simulink model "zero_moment_direction_ctrl"  (R2018b)
settings: Solver=VariableStepAuto  StartTime=0.0  StopTime=40  RelTol=1e-3
values from neighbouring files (symbols this model uses):
  alpha_0 = alpha    (= 0.237364778271)    [IdealParameter.m]    (also in Parameter.m = alpha; ParameterIdeal.m = alpha*1.01; ParameterVIVE.m = alpha*1.01; ParameterVO.m = alpha*1.01)
  angular_noise = 0    [IdealParameter.m]    (also in Parameter.m = 0.5; ParameterIdeal.m; ParameterVIVE.m; ParameterVO.m)
  b_0 = b*1.15    (= 1.265e-06)    [IdealParameter.m]    (also in Parameter.m = 8.944e-07; ParameterIdeal.m; ParameterVIVE.m; ParameterVO.m)
  beta_0 = beta    (= 0)    [IdealParameter.m]    (also in Parameter.m = beta; ParameterIdeal.m = beta*0.99; ParameterVIVE.m = beta*0.99; ParameterVO.m = beta*0.99)
  g_0 = g*0.99    (= 9.7119)    [IdealParameter.m]    (also in Parameter.m = 9.81; ParameterIdeal.m = 9.81; ParameterVIVE.m = 9.81; ParameterVO.m = 9.81)
  IB = [Ixx 0 0; 0 Iyy 0; 0 0 Izz]    [IdealParameter.m]    (also in ParLuk11.m; Parameter.m; ParameterIdeal.m; ParameterVIVE.m)
  IB_0 = IB*1.07    [IdealParameter.m]    (also in Parameter.m = IB; ParameterIdeal.m; ParameterVIVE.m; ParameterVO.m)
  K_0 = Ts/(T_rotor_0+Ts)    (= 0.0384615384615)    [IdealParameter.m]    (also in Parameter.m; ParameterIdeal.m; ParameterVIVE.m = 0.0350877192982; ParameterVO.m = 0.214285714286)
  k_0 = k*1.16    (= 6.496e-05)    [IdealParameter.m]    (also in Parameter.m = 4.472e-05; ParameterIdeal.m; ParameterVIVE.m = 5.9508e-05; ParameterVO.m)
  K_ad = 4    [Parameter.m]
  K_ap = 2    [Parameter.m]
  K_pd = 8    [Parameter.m]
  K_pp = 6    [Parameter.m]
  K_z = 5    [Parameter.m]
  L_0 = L*1.02    (= 0.408)    [IdealParameter.m]    (also in Parameter.m = 0.4; ParameterIdeal.m; ParameterVIVE.m = 0.612; ParameterVO.m)
  m_0 = m*1.03    (= 2.575)    [IdealParameter.m]    (also in Parameter.m = 4.85; ParameterIdeal.m = 4.9955; ParameterVIVE.m = 4.52994; ParameterVO.m = 4.9955)
  omega_noise = 0    [IdealParameter.m]    (also in Parameter.m = 0.0027; ParameterIdeal.m; ParameterVIVE.m; ParameterVO.m)
  p_noise = 0    [IdealParameter.m]    (also in Parameter.m = 0.00064; ParameterIdeal.m; ParameterVIVE.m; ParameterVO.m)
  rot_vel_max = (6300 * pi/30)^2    (= 435249.554088)    [Parameter.m]    (also in ParameterVIVE.m = 356292.718879; Parameter_old.m)
  rot_vel_min = 0    [Parameter.m]    (also in ParameterVIVE.m; Parameter_old.m)
  T_delay = 0    [IdealParameter.m]    (also in Parameter.m = 0.04; ParameterIdeal.m; ParameterVIVE.m = 0.04; ParameterVO.m = 0.1)
  T_rotor = 0.1    [IdealParameter.m]    (also in Parameter.m; ParameterIdeal.m; ParameterVIVE.m; ParameterVO.m)
  Ts = 1/250    (= 0.004)    [IdealParameter.m]    (also in Parameter.m; ParameterIdeal.m; ParameterVIVE.m; ParameterVO.m = 0.03)
  v_noise = 0    [IdealParameter.m]    (also in Parameter.m = 0.0014; ParameterIdeal.m; ParameterVIVE.m; ParameterVO.m)
  z_p_0 = T_rotor_0/(T_rotor_0+Ts)    (= 0.961538461538)    [IdealParameter.m]    (also in Parameter.m; ParameterIdeal.m; ParameterVIVE.m = 0.964912280702; ParameterVO.m = 0.785714285714)
libraries: simulink x7, vrlib x2
settings Model: Creator=HaloCao  LastModifiedBy=HaloCao

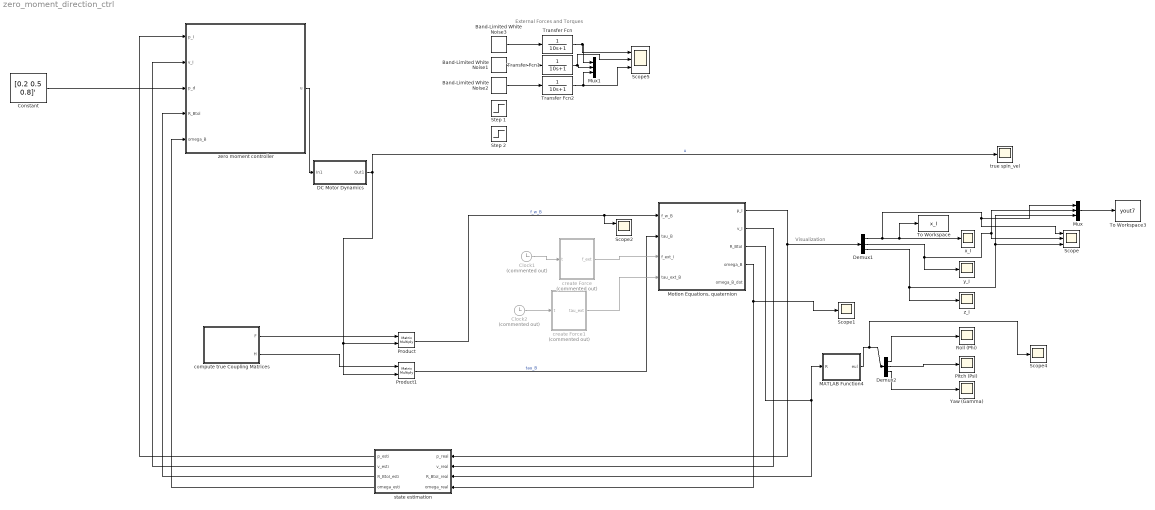
== system zero_moment_direction_ctrl ==
  note: Visualization
  note: External Forces and Torques
  Band-Limited White Noise1 : simulink/Sources/Band-Limited White Noise  Cov=1  Ts=0.1  seed=[23342]  VectorParams1D=off
  Band-Limited White Noise2 : simulink/Sources/Band-Limited White Noise  Cov=1  Ts=0.1  seed=[23441]  VectorParams1D=off
  Band-Limited White Noise3 : simulink/Sources/Band-Limited White Noise  Cov=1  Ts=0.1  seed=[23342]  VectorParams1D=off
  Clock1 : Clock  Commented=on
  Clock2 : Clock  Commented=on
  Constant : Constant  Value="[0.2  0.5 0.8]'"
  "DC Motor Dynamics " : Subsystem  TreatAsAtomicUnit=on
  Demux1 : Demux  Outputs=3
  Demux2 : Demux  Outputs=3
  MATLAB Function4 : MATLAB Function  TreatAsAtomicUnit=on
  "Motion Equations, quaternion" : Subsystem
  Mux : Mux  Inputs=3
  Mux1 : Mux  Inputs=3
  Pitch (Psi) : Scope
  Product : Product  Multiplication=Matrix(*)
  Product1 : Product  Multiplication=Matrix(*)
  Roll (Phi) : Scope
  Scope : Scope  NumInputPorts=3
  Scope1 : Scope
  Scope2 : Scope  NumInputPorts=2
  Scope4 : Scope
  Scope5 : Scope  NumInputPorts=3
  Step 1 : Step  Before=[0;0;0]  After=[10;1;1]  SampleTime=0  VectorParams1D=off
  Step 2 : Step  Before=[0;0;0]  After=[5;1;1]  SampleTime=0  VectorParams1D=off
  To Workspace : ToWorkspace  VariableName=x_I  SaveFormat=Timeseries  SampleTime=-1
  To Workspace3 : ToWorkspace  VariableName=yout7  SampleTime=-1
      settings: Save2DSignal=2-D array (concatenate along first dimension)
  Transfer Fcn : TransferFcn  Denominator=[10 1]
  Transfer Fcn1 : TransferFcn  Denominator=[10 1]
  Transfer Fcn2 : TransferFcn  Denominator=[10 1]
  Yaw (Gamma) : Scope
  compute true Coupling Matrices : Subsystem
  create Force : MATLAB Function  Commented=on  TreatAsAtomicUnit=on
  create Force1 : MATLAB Function  Commented=on  TreatAsAtomicUnit=on
  state estimation : Subsystem
  true spin_vel : Scope
  x_I : Scope
  y_I : Scope
  z_I : Scope
  zero moment controller : Subsystem
  wires:
  zero moment controller/1(u) -> "DC Motor Dynamics "/1(In1)
  "Motion Equations, quaternion"/1(p_I) -> state estimation/1(p_real), Demux1/1
  Demux2/2 -> Pitch (Psi)/1
  Demux1/2 -> Mux/2, Scope/2, y_I/1
  Product1/1 -> "Motion Equations, quaternion"/2(tau_B)  "tau_B"
  Demux2/3 -> Yaw (Gamma)/1
  "Motion Equations, quaternion"/2(v_I) -> state estimation/2(v_real)
  MATLAB Function4/1(eul) -> Scope4/1, Demux2/1
  Demux1/3 -> Mux/3, Scope/3, z_I/1
  "Motion Equations, quaternion"/4(omega_B) -> state estimation/4(omega_real), Scope1/1
  Demux2/1 -> Roll (Phi)/1
  "Motion Equations, quaternion"/3(R_BtoI) -> state estimation/3(R_BtoI_real), MATLAB Function4/1(R)
  Constant/1 -> zero moment controller/3(p_d)
  Demux1/1 -> Mux/1, Scope/1, To Workspace/1, x_I/1
  Clock1/1 -> create Force/1(t)
  compute true Coupling Matrices/1(F) -> Product/1
  compute true Coupling Matrices/2(H) -> Product1/1
  "DC Motor Dynamics "/1(Out1) -> Product1/2, Product/2, true spin_vel/1  "u"
  Product/1 -> Scope2/1, "Motion Equations, quaternion"/1("f_w_B ")  "f_w_B"
  Mux/1 -> To Workspace3/1
  state estimation/3(R_BtoI_esti) -> zero moment controller/4(R_Btol)
  state estimation/4(omega_esti) -> zero moment controller/5(omega_B)
  state estimation/2(v_esti) -> zero moment controller/2(v_I)
  state estimation/1(p_esti) -> zero moment controller/1(p_I)
  Clock2/1 -> create Force1/1(t)
  Transfer Fcn1/1 -> Scope5/2, Mux1/2
  Band-Limited White Noise3/1 -> Transfer Fcn/1
  Transfer Fcn2/1 -> Scope5/3, Mux1/3
  Band-Limited White Noise2/1 -> Transfer Fcn2/1
  Band-Limited White Noise1/1 -> Transfer Fcn1/1
  Transfer Fcn/1 -> Scope5/1, Mux1/1
  create Force1/1(tau_ext) -> "Motion Equations, quaternion"/4(tau_ext_B)
  create Force/1(f_ext) -> "Motion Equations, quaternion"/3(f_ext_I)

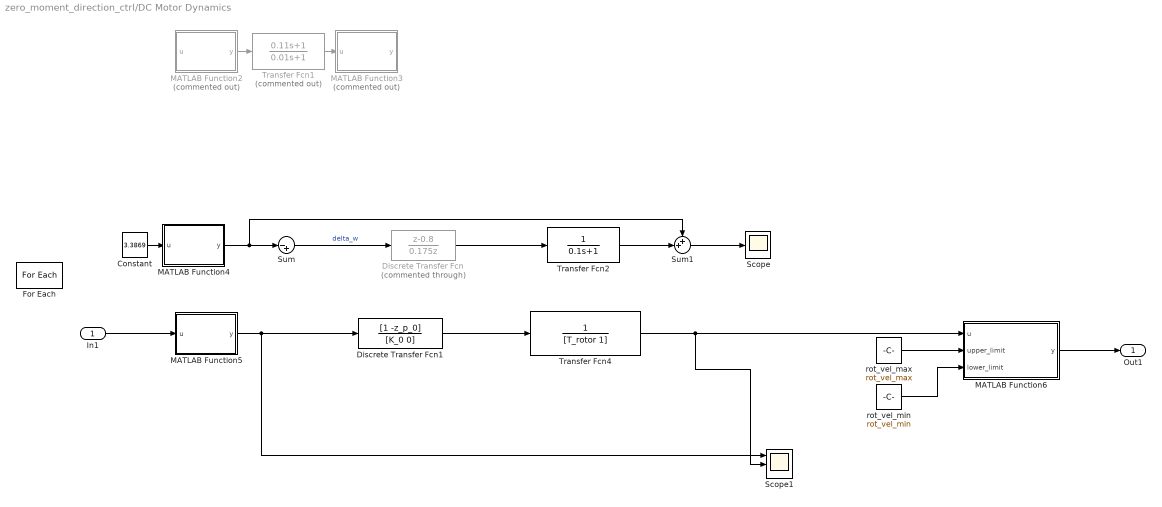
== system zero_moment_direction_ctrl/DC Motor Dynamics  ==
  In1 : Inport  Partition=on  PartitionDimension=1  PartitionWidth=1  PartitionOffset=0
  Constant : Constant  Value=3.3869
  Discrete Transfer Fcn : DiscreteTransferFcn  Commented=through  Numerator=[1 -0.8]  Denominator=[0.175 0]  SampleTime=Ts
  Discrete Transfer Fcn1 : DiscreteTransferFcn  Numerator=[1 -z_p_0]  Denominator=[K_0 0]  InitialStates=274  SampleTime=Ts
  For Each : ForEach  DisableCoverage=on  IndexMode=One-based
  MATLAB Function2 : MATLAB Function  Commented=on  TreatAsAtomicUnit=on
  MATLAB Function3 : MATLAB Function  Commented=on  TreatAsAtomicUnit=on
  MATLAB Function4 : MATLAB Function  TreatAsAtomicUnit=on
  MATLAB Function5 : MATLAB Function  TreatAsAtomicUnit=on  SystemSampleTime=Ts
  MATLAB Function6 : MATLAB Function  TreatAsAtomicUnit=on
  Scope : Scope
  Scope1 : Scope  NumInputPorts=3
  Sum : Sum  Inputs=|-+
  Sum1 : Sum  Inputs=++|
  Transfer Fcn1 : TransferFcn  Commented=on  Numerator=[0.11 1]  Denominator=[0.01 1]
  Transfer Fcn2 : TransferFcn  Denominator=[0.1 1]
  Transfer Fcn4 : TransferFcn  Denominator=[T_rotor 1]
  rot_vel_max : Constant  Value=rot_vel_max
  rot_vel_min : Constant  Value=rot_vel_min
  Out1 : Outport  ConcatenationDimension=1
  wires:
  Transfer Fcn1/1 -> MATLAB Function3/1(u)
  MATLAB Function2/1(y) -> Transfer Fcn1/1
  Constant/1 -> MATLAB Function4/1(u)
  MATLAB Function4/1(y) -> Sum1/1, Sum/1
  Sum/1 -> Discrete Transfer Fcn/1  "delta_w"
  In1/1 -> MATLAB Function5/1(u)
  MATLAB Function5/1(y) -> Discrete Transfer Fcn1/1, Scope1/1
  Discrete Transfer Fcn/1 -> Transfer Fcn2/1
  Transfer Fcn2/1 -> Sum1/2
  MATLAB Function6/1(y) -> Out1/1
  Sum1/1 -> Scope/1
  Discrete Transfer Fcn1/1 -> Transfer Fcn4/1
  Transfer Fcn4/1 -> Scope1/2, MATLAB Function6/1(u)
  rot_vel_max/1 -> MATLAB Function6/2(upper_limit)
  rot_vel_min/1 -> MATLAB Function6/3(lower_limit)

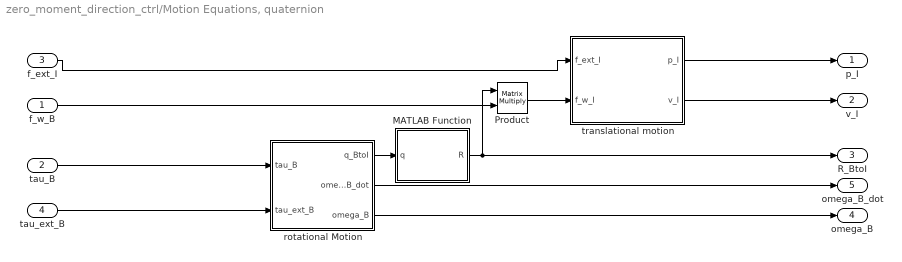
== system zero_moment_direction_ctrl/Motion Equations, quaternion ==
  "f_w_B " : Inport
  tau_B : Inport  Port=2
  f_ext_I : Inport  Port=3
  tau_ext_B : Inport  Port=4
  MATLAB Function : MATLAB Function  TreatAsAtomicUnit=on
  Product : Product  Multiplication=Matrix(*)
  rotational Motion : Subsystem
  translational motion : Subsystem
  p_I : Outport
  v_I : Outport  Port=2
  R_BtoI : Outport  Port=3
  omega_B : Outport  Port=4
  omega_B_dot : Outport  Port=5
  wires:
  f_ext_I/1 -> translational motion/1(f_ext_I)
  translational motion/1(p_I) -> p_I/1
  translational motion/2(v_I) -> v_I/1
  Product/1 -> translational motion/2(f_w_I)
  tau_B/1 -> rotational Motion/1(tau_B)
  tau_ext_B/1 -> rotational Motion/2(tau_ext_B)
  rotational Motion/2(omega_B_dot) -> omega_B_dot/1
  rotational Motion/3(omega_B) -> omega_B/1
  "f_w_B "/1 -> Product/2
  rotational Motion/1(q_BtoI) -> MATLAB Function/1(q)
  MATLAB Function/1(R) -> Product/1, R_BtoI/1

== system zero_moment_direction_ctrl/compute true Coupling Matrices ==
  Constant : Constant  Value=alpha_0
  Constant2 : Constant  Value=beta_0
  Constant3 : Constant  Value=k_0
  Constant4 : Constant  Value=L_0
  Constant5 : Constant  Value=b_0
  MATLAB Function5 : MATLAB Function  TreatAsAtomicUnit=on
  MATLAB Function6 : MATLAB Function  TreatAsAtomicUnit=on
  F : Outport
  H : Outport  Port=2
  wires:
  MATLAB Function5/6(e_r6) -> MATLAB Function6/6(e_r6)
  Constant4/1 -> MATLAB Function6/9(L)
  MATLAB Function5/2(e_r2) -> MATLAB Function6/2(e_r2)
  MATLAB Function5/3(e_r3) -> MATLAB Function6/3(e_r3)
  MATLAB Function5/4(e_r4) -> MATLAB Function6/4(e_r4)
  MATLAB Function5/1(e_r1) -> MATLAB Function6/1(e_r1)
  MATLAB Function5/5(e_r5) -> MATLAB Function6/5(e_r5)
  Constant3/1 -> MATLAB Function6/8(k)
  Constant2/1 -> MATLAB Function5/2(beta)
  Constant/1 -> MATLAB Function5/1(alpha)
  Constant5/1 -> MATLAB Function6/7(b)
  MATLAB Function6/2(H) -> H/1
  MATLAB Function6/1(F) -> F/1

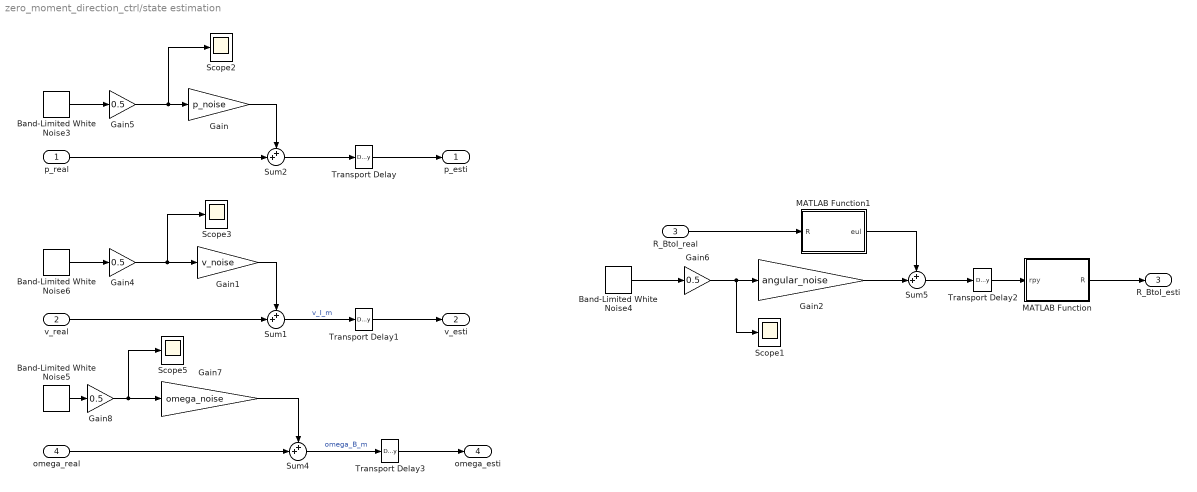
== system zero_moment_direction_ctrl/state estimation ==
  p_real : Inport
  v_real : Inport  Port=2
  R_BtoI_real : Inport  Port=3
  omega_real : Inport  Port=4
  Band-Limited White Noise3 : simulink/Sources/Band-Limited White Noise  Cov=[0.01; 0.01; 0.01]  Ts=Ts  seed=[22352; 29655; 12541]  VectorParams1D=off
  Band-Limited White Noise4 : simulink/Sources/Band-Limited White Noise  Cov=[0.01; 0.01; 0.01]  Ts=Ts  seed=[11351; 22653; 52546]  VectorParams1D=off
  Band-Limited White Noise5 : simulink/Sources/Band-Limited White Noise  Cov=[0.01; 0.01; 0.01]  Ts=Ts  seed=[12451; 82653; 82546]  VectorParams1D=off
  Band-Limited White Noise6 : simulink/Sources/Band-Limited White Noise  Cov=[0.01; 0.01; 0.01]  Ts=Ts  seed=[22351; 29653; 12546]  VectorParams1D=off
  Gain : Gain  Gain=p_noise
  Gain1 : Gain  Gain=v_noise
  Gain2 : Gain  Gain=angular_noise
  Gain{4..6,8} (4 alike) : Gain  Gain=0.5
  Gain7 : Gain  Gain=omega_noise
  MATLAB Function : MATLAB Function  TreatAsAtomicUnit=on
  MATLAB Function1 : MATLAB Function  TreatAsAtomicUnit=on
  Scope{1..3,5} (4 alike) : Scope
  Sum{1..2,4..5} (4 alike) : Sum  Inputs=++|
  Transport Delay{,1..3} (4 alike) : TransportDelay  DelayTime=T_delay  InitialOutput=[0;0;0]
  p_esti : Outport
  v_esti : Outport  Port=2
  R_BtoI_esti : Outport  Port=3
  omega_esti : Outport  Port=4
  wires:
  R_BtoI_real/1 -> MATLAB Function1/1(R)
  p_real/1 -> Sum2/2
  Transport Delay/1 -> p_esti/1
  Sum4/1 -> Transport Delay3/1  "omega_B_m"
  Gain/1 -> Sum2/1
  Gain1/1 -> Sum1/1
  Sum2/1 -> Transport Delay/1
  Sum1/1 -> Transport Delay1/1  "v_I_m"
  MATLAB Function1/1(eul) -> Sum5/1
  Sum5/1 -> Transport Delay2/1
  Gain2/1 -> Sum5/2
  Transport Delay2/1 -> MATLAB Function/1(rpy)
  v_real/1 -> Sum1/2
  omega_real/1 -> Sum4/2
  MATLAB Function/1(R) -> R_BtoI_esti/1
  Transport Delay1/1 -> v_esti/1
  Gain5/1 -> Scope2/1, Gain/1
  Band-Limited White Noise3/1 -> Gain5/1
  Gain4/1 -> Gain1/1, Scope3/1
  Band-Limited White Noise6/1 -> Gain4/1
  Band-Limited White Noise5/1 -> Gain8/1
  Gain8/1 -> Scope5/1, Gain7/1
  Gain6/1 -> Scope1/1, Gain2/1
  Band-Limited White Noise4/1 -> Gain6/1
  Transport Delay3/1 -> omega_esti/1
  Gain7/1 -> Sum4/1

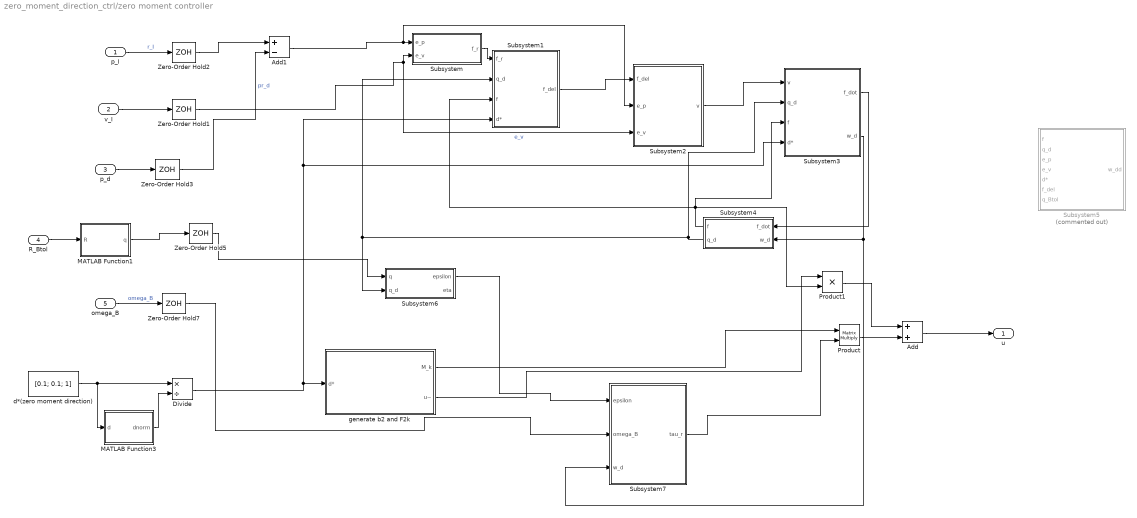
== system zero_moment_direction_ctrl/zero moment controller ==
  p_I : Inport
  v_I : Inport  Port=2
  p_d : Inport  Port=3
  R_Btol : Inport  Port=4
  omega_B : Inport  Port=5
  Add : Sum
  Add1 : Sum  Inputs=+-
  Divide : Product  Inputs=*/
  MATLAB Function1 : MATLAB Function  TreatAsAtomicUnit=on
  MATLAB Function3 : MATLAB Function  TreatAsAtomicUnit=on
  Product : Product  Multiplication=Matrix(*)
  Product1 : Product
  Subsystem : Subsystem
  Subsystem1 : Subsystem
  Subsystem2 : Subsystem
  Subsystem3 : Subsystem
  Subsystem4 : Subsystem
  Subsystem5 : Subsystem  Commented=on
  Subsystem6 : Subsystem
  Subsystem7 : Subsystem
  Zero-Order Hold{1..3,5,7} (5 alike) : ZeroOrderHold  SampleTime=Ts
  d*(zero moment direction) : Constant  Value=[0.1; 0.1; 1]
  generate b2 and F2k : Subsystem
  u : Outport
  wires:
  p_d/1 -> Zero-Order Hold3/1
  p_I/1 -> Zero-Order Hold2/1  "r_I"
  Zero-Order Hold5/1 -> Subsystem6/1(q)
  omega_B/1 -> Zero-Order Hold7/1  "omega_B"
  Zero-Order Hold1/1 -> Subsystem/2(e_v), Subsystem2/3(e_v)  "e_v"
  Subsystem/1(f_r) -> Subsystem1/1(f_r)
  Subsystem1/1(f_del) -> Subsystem2/1(f_del)
  Subsystem2/1(v) -> Subsystem3/1(v)
  Subsystem3/1(f_dot) -> Subsystem4/1(f_dot)
  Subsystem3/2(w_d) -> Subsystem7/3(w_d), Subsystem4/2(w_d)
  Subsystem4/1(f) -> Subsystem3/3(f), Product1/2, Subsystem1/3(f)
  Subsystem7/1(tau_r) -> Product/2
  generate b2 and F2k/1(M_k) -> Product/1
  Add/1 -> u/1
  generate b2 and F2k/2(u~) -> Product1/1
  Product/1 -> Add/2
  Product1/1 -> Add/1
  Subsystem6/1(epsilon) -> Subsystem7/1(epsilon)
  v_I/1 -> Zero-Order Hold1/1
  Zero-Order Hold3/1 -> Add1/2  "pr_d"
  Zero-Order Hold2/1 -> Add1/1
  MATLAB Function3/1(dnorm) -> Divide/2
  d*(zero moment direction)/1 -> MATLAB Function3/1(d), Divide/1
  Divide/1 -> Subsystem3/4(d*), Subsystem1/4(d*), generate b2 and F2k/1(d*)
  Add1/1 -> Subsystem2/2(e_p), Subsystem/1(e_p)
  Subsystem4/2(q_d) -> Subsystem1/2(q_d), Subsystem6/2(q_d), Subsystem3/2(q_d)
  Zero-Order Hold7/1 -> Subsystem7/2(omega_B)
  R_Btol/1 -> MATLAB Function1/1(R)
  MATLAB Function1/1(q) -> Zero-Order Hold5/1

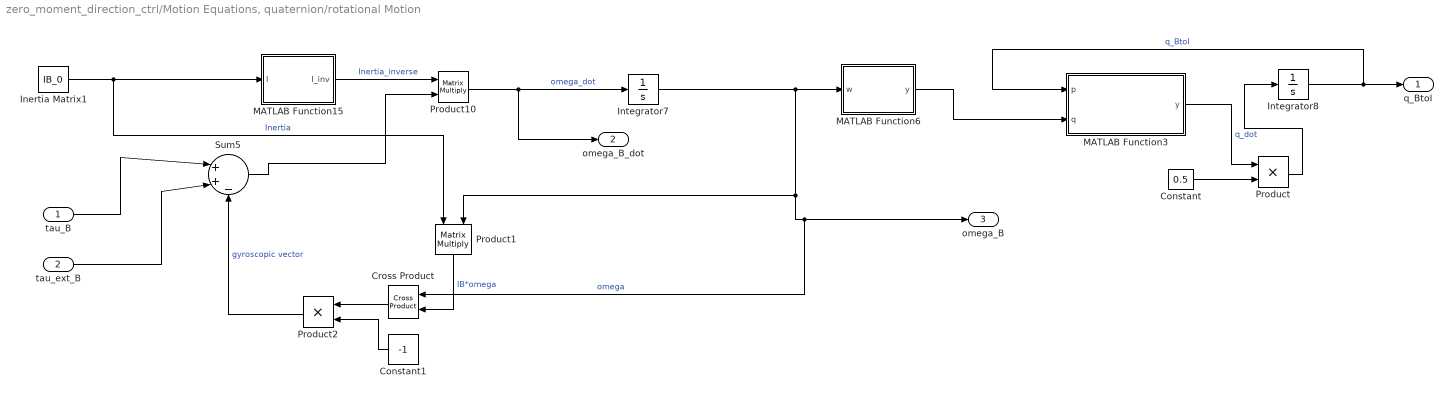
== system zero_moment_direction_ctrl/Motion Equations, quaternion/rotational Motion ==
  tau_B : Inport
  tau_ext_B : Inport  Port=2
  Constant : Constant  Value=0.5
  Constant1 : Constant  Value=-1
  Cross Product : vrlib/Utilities/Cross Product
      settings: SourceProductBaseCode=VR
  Inertia Matrix1 : Constant  Value=IB_0  VectorParams1D=off
  Integrator7 : Integrator  InitialCondition=[0 0 0]'
  Integrator8 : Integrator  InitialCondition=[0 0 0 1]'
  MATLAB Function15 : MATLAB Function  TreatAsAtomicUnit=on
  MATLAB Function3 : MATLAB Function  TreatAsAtomicUnit=on
  MATLAB Function6 : MATLAB Function  TreatAsAtomicUnit=on
  Product : Product
  Product1 : Product  Multiplication=Matrix(*)
  Product10 : Product  Multiplication=Matrix(*)
  Product2 : Product
  Sum5 : Sum  Inputs=|++-
  q_BtoI : Outport
  omega_B_dot : Outport  Port=2
  omega_B : Outport  Port=3
  wires:
  Product10/1 -> omega_B_dot/1, Integrator7/1  "omega_dot"
  tau_B/1 -> Sum5/1
  Integrator7/1 -> Product1/2, Cross Product/1, omega_B/1, MATLAB Function6/1(w)  "omega"
  tau_ext_B/1 -> Sum5/2
  Inertia Matrix1/1 -> Product1/1, MATLAB Function15/1(I)  "Inertia"
  Sum5/1 -> Product10/2
  MATLAB Function15/1(I_inv) -> Product10/1  "Inertia_inverse"
  Integrator8/1 -> MATLAB Function3/1(p), q_BtoI/1  "q_BtoI"
  Product2/1 -> Sum5/3  "gyroscopic vector"
  Product1/1 -> Cross Product/2  "IB*omega"
  Constant/1 -> Product/2
  Product/1 -> Integrator8/1
  MATLAB Function3/1(y) -> Product/1  "q_dot"
  MATLAB Function6/1(y) -> MATLAB Function3/2(q)
  Cross Product/1 -> Product2/1
  Constant1/1 -> Product2/2

== system zero_moment_direction_ctrl/Motion Equations, quaternion/translational motion ==
  f_ext_I : Inport
  f_w_I : Inport  Port=2
  Constant1 : Constant  Value=[0 0 g_0]'  VectorParams1D=off
  Gain1 : Gain  Gain=m_0
  Gain4 : Gain  Gain=1/m_0
  Integrator2 : Integrator  InitialCondition=[0;0;0]
  Integrator3 : Integrator  InitialCondition=[0 0 0]'
  Sum : Sum  Inputs=++-
  p_I : Outport
  v_I : Outport  Port=2
  wires:
  Sum/1 -> Gain4/1
  f_ext_I/1 -> Sum/1
  Gain4/1 -> Integrator2/1  "a_I"
  Integrator2/1 -> v_I/1, Integrator3/1  "v_I"
  Gain1/1 -> Sum/3  "gravity"
  Constant1/1 -> Gain1/1
  Integrator3/1 -> p_I/1  "p_I"
  f_w_I/1 -> Sum/2

== system zero_moment_direction_ctrl/zero moment controller/Subsystem ==
  e_p : Inport
  e_v : Inport  Port=2
  Constant1 : Constant  Value=[0 0 g_0]'  VectorParams1D=off
  Gain1 : Gain  Gain=m_0
  K_pd : Constant  Value=K_pd
  K_pp : Constant  Value=K_pp
  Product : Product
  Product1 : Product
  Sum : Sum  Inputs=-+-
  f_r : Outport
  wires:
  Product/1 -> Sum/1
  Constant1/1 -> Gain1/1
  Gain1/1 -> Sum/2  "gravity"
  K_pp/1 -> Product/1
  e_p/1 -> Product/2
  K_pd/1 -> Product1/1
  e_v/1 -> Product1/2
  Product1/1 -> Sum/3
  Sum/1 -> f_r/1

== system zero_moment_direction_ctrl/zero moment controller/Subsystem1 ==
  f_r : Inport
  q_d : Inport  Port=2
  f : Inport  Port=3
  d* : Inport  Port=4
  MATLAB Function1 : MATLAB Function  TreatAsAtomicUnit=on
  Minus : Sum  Inputs=-+
  Product : Product  Multiplication=Matrix(*)
  Product1 : Product
  f_del : Outport
  wires:
  d*/1 -> Product/2
  Product/1 -> Product1/1
  f/1 -> Product1/2
  Product1/1 -> Minus/2
  f_r/1 -> Minus/1
  Minus/1 -> f_del/1
  MATLAB Function1/1(R) -> Product/1
  q_d/1 -> MATLAB Function1/1(q)

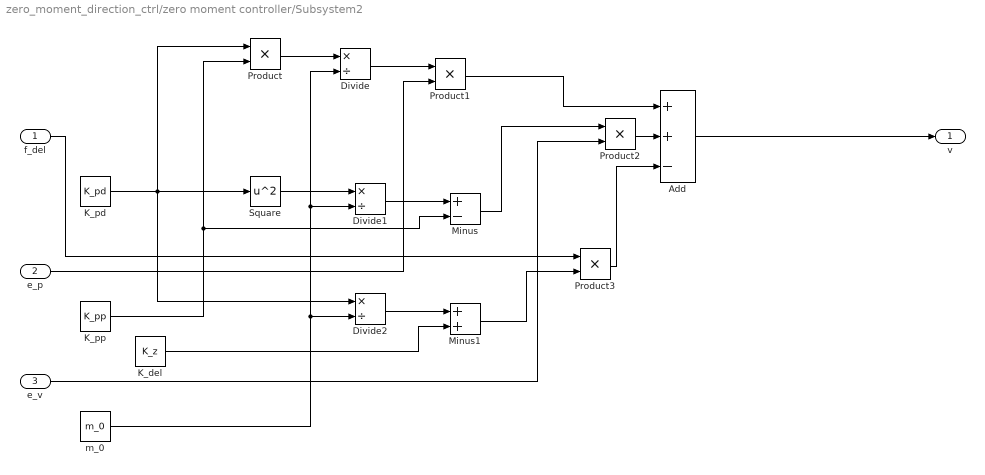
== system zero_moment_direction_ctrl/zero moment controller/Subsystem2 ==
  f_del : Inport
  e_p : Inport  Port=2
  e_v : Inport  Port=3
  Add : Sum  Inputs=++-
  Divide : Product  Inputs=*/
  Divide1 : Product  Inputs=*/
  Divide2 : Product  Inputs=*/
  K_del : Constant  Value=K_z
  K_pd : Constant  Value=K_pd
  K_pp : Constant  Value=K_pp
  Minus : Sum  Inputs=+-
  Minus1 : Sum
  Product{,1..3} (4 alike) : Product
  Square : Math  Operator=square  SaturateOnIntegerOverflow=on
  m_0 : Constant  Value=m_0
  v : Outport
  wires:
  K_pd/1 -> Product/1, Divide2/1, Square/1
  K_pp/1 -> Minus/2, Product/2
  Product/1 -> Divide/1
  m_0/1 -> Divide2/2, Divide1/2, Divide/2
  Divide/1 -> Product1/1
  e_p/1 -> Product1/2
  Product1/1 -> Add/1
  Square/1 -> Divide1/1
  Divide1/1 -> Minus/1
  Minus/1 -> Product2/1
  e_v/1 -> Product2/2
  Product2/1 -> Add/2
  Divide2/1 -> Minus1/1
  K_del/1 -> Minus1/2
  Product3/1 -> Add/3
  Minus1/1 -> Product3/2
  f_del/1 -> Product3/1
  Add/1 -> v/1

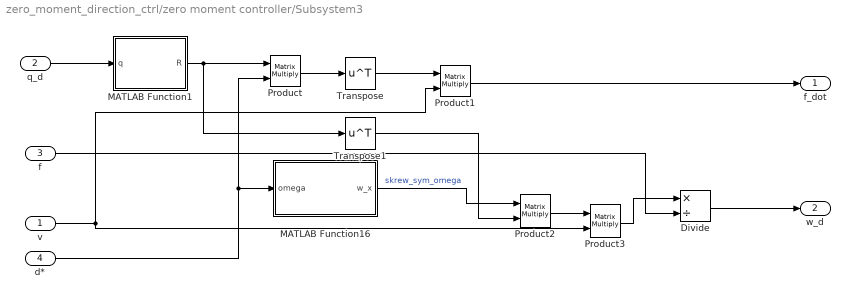
== system zero_moment_direction_ctrl/zero moment controller/Subsystem3 ==
  v : Inport
  q_d : Inport  Port=2
  f : Inport  Port=3
  d* : Inport  Port=4
  Divide : Product  Inputs=*/
  MATLAB Function1 : MATLAB Function  TreatAsAtomicUnit=on
  MATLAB Function16 : MATLAB Function  TreatAsAtomicUnit=on
  Product{,1..3} (4 alike) : Product  Multiplication=Matrix(*)
  Transpose : Math  Operator=transpose  SaturateOnIntegerOverflow=on
  Transpose1 : Math  Operator=transpose  SaturateOnIntegerOverflow=on
  f_dot : Outport
  w_d : Outport  Port=2
  wires:
  d*/1 -> Product/2, MATLAB Function16/1(omega)
  Product/1 -> Transpose/1
  Transpose/1 -> Product1/1
  v/1 -> Product1/2, Product3/2
  Product1/1 -> f_dot/1
  f/1 -> Divide/2
  Divide/1 -> w_d/1
  MATLAB Function16/1(w_x) -> Product2/1  "skrew_sym_omega"
  Transpose1/1 -> Product2/2
  q_d/1 -> MATLAB Function1/1(q)
  MATLAB Function1/1(R) -> Transpose1/1, Product/1
  Product2/1 -> Product3/1
  Product3/1 -> Divide/1

== system zero_moment_direction_ctrl/zero moment controller/Subsystem4 ==
  f_dot : Inport
  w_d : Inport  Port=2
  Constant : Constant  Value=0.5
  Integrator : Integrator  InitialCondition=47.5
  Integrator1 : Integrator  InitialCondition=[0 0 0 1]'
  MATLAB Function : MATLAB Function  TreatAsAtomicUnit=on
  MATLAB Function1 : MATLAB Function  TreatAsAtomicUnit=on
  Product : Product
  f : Outport
  q_d : Outport  Port=2
  wires:
  Integrator/1 -> f/1
  Integrator1/1 -> MATLAB Function/1(p), q_d/1
  w_d/1 -> MATLAB Function1/1(w)
  MATLAB Function/1(y) -> Product/1
  Constant/1 -> Product/2
  MATLAB Function1/1(y) -> MATLAB Function/2(q)
  f_dot/1 -> Integrator/1
  Product/1 -> Integrator1/1

== system zero_moment_direction_ctrl/zero moment controller/Subsystem5 ==
  f : Inport
  q_d : Inport  Port=2
  e_p : Inport  Port=3
  e_v : Inport  Port=4
  d* : Inport  Port=5
  f_del : Inport  Port=6
  q_Btol : Inport  Port=7
  MATLAB Function : MATLAB Function  TreatAsAtomicUnit=on
  Product2 : Product  Multiplication=Matrix(*)
  teil1 : Subsystem
  teil2 : Subsystem
  w_dd : Outport
  wires:
  q_d/1 -> teil2/2(q_d), teil1/2(q_d)
  f/1 -> teil2/1(f), teil1/1(f)
  d*/1 -> teil1/3(d*), teil2/5(d*)
  teil1/1(Out1) -> Product2/1
  f_del/1 -> teil2/6(f_del)
  e_p/1 -> teil2/3(e_p)
  e_v/1 -> teil2/4(e_v)
  Product2/1 -> w_dd/1
  teil2/1(Teil2) -> Product2/2
  q_Btol/1 -> MATLAB Function/1(q)
  MATLAB Function/1(R) -> teil2/7(R_Btol)

== system zero_moment_direction_ctrl/zero moment controller/Subsystem6 ==
  q : Inport
  q_d : Inport  Port=2
  MATLAB Function : MATLAB Function  TreatAsAtomicUnit=on
  MATLAB Function1 : MATLAB Function  TreatAsAtomicUnit=on
  MATLAB Function2 : MATLAB Function  TreatAsAtomicUnit=on
  epsilon : Outport
  eta : Outport  Port=2
  wires:
  q/1 -> MATLAB Function1/2(q)
  q_d/1 -> MATLAB Function/1(q)
  MATLAB Function/1(y) -> MATLAB Function1/1(p)
  MATLAB Function1/1(y) -> MATLAB Function2/1(q)
  MATLAB Function2/1(epsilon) -> epsilon/1
  MATLAB Function2/2(eta) -> eta/1

== system zero_moment_direction_ctrl/zero moment controller/Subsystem7 ==
  epsilon : Inport
  omega_B : Inport  Port=2
  w_d : Inport  Port=3
  Cross Product : vrlib/Utilities/Cross Product
      settings: SourceProductBaseCode=VR
  Inertia Matrix1 : Constant  Value=IB  VectorParams1D=off
  K_ad : Constant  Value=K_ad
  K_ap : Constant  Value=K_ap
  Minus : Sum  Inputs=--+
  Minus1 : Sum  Inputs=-+
  Product : Product
  Product1 : Product
  Product3 : Product  Multiplication=Matrix(*)
  tau_r : Outport
  wires:
  K_ap/1 -> Product/1
  epsilon/1 -> Product/2
  Product/1 -> Minus/1
  K_ad/1 -> Product1/1
  omega_B/1 -> Product3/2, Cross Product/1, Minus1/2
  Minus1/1 -> Product1/2
  Product1/1 -> Minus/2
  Inertia Matrix1/1 -> Product3/1  "Inertia"
  Product3/1 -> Cross Product/2
  Cross Product/1 -> Minus/3
  w_d/1 -> Minus1/1
  Minus/1 -> tau_r/1

== system zero_moment_direction_ctrl/zero moment controller/generate b2 and F2k ==
  d* : Inport
  Divide : Product  Inputs=*/
  MATLAB Function : MATLAB Function  TreatAsAtomicUnit=on
  MATLAB Function1 : MATLAB Function  TreatAsAtomicUnit=on
  MATLAB Function2 : MATLAB Function  TreatAsAtomicUnit=on
  MATLAB Function3 : MATLAB Function  TreatAsAtomicUnit=on
  Vup : Constant  Value=[1 42 70 10 13 16; 2 5 83 11 14 17; 34 6 9 1 15 18]
  compute true Coupling Matrices : Subsystem
  M_k : Outport
  u~ : Outport  Port=2
  wires:
  compute true Coupling Matrices/2(H) -> MATLAB Function1/2(M), MATLAB Function/2(H)
  compute true Coupling Matrices/1(F) -> MATLAB Function2/1(F), MATLAB Function/1(F)
  Vup/1 -> MATLAB Function2/2(Vup)
  MATLAB Function1/1(M_k) -> M_k/1
  MATLAB Function/1(b2) -> u~/1
  MATLAB Function2/1(V) -> MATLAB Function1/1(V)
  d*/1 -> Divide/1, MATLAB Function3/1(d)
  MATLAB Function3/1(dnorm) -> Divide/2
  Divide/1 -> MATLAB Function/3(d)

== system zero_moment_direction_ctrl/zero moment controller/Subsystem5/teil1 ==
  note: Teil 1
  f : Inport
  q_d : Inport  Port=2
  d* : Inport  Port=3
  Divide : Product  Inputs=*/
  MATLAB Function : MATLAB Function  Commented=through  TreatAsAtomicUnit=on
  MATLAB Function1 : MATLAB Function  TreatAsAtomicUnit=on
  MATLAB Function2 : MATLAB Function  TreatAsAtomicUnit=on
  Product : Product  Multiplication=Matrix(*)
  Transpose : Math  Operator=transpose  SaturateOnIntegerOverflow=on
  Out1 : Outport
  wires:
  f/1 -> Divide/2
  Product/1 -> Divide/1
  Divide/1 -> Out1/1
  d*/1 -> MATLAB Function1/1(omega)
  MATLAB Function1/1(w_x) -> Product/1  "skrew_sym_omega"
  Transpose/1 -> Product/2
  MATLAB Function2/1(R) -> Transpose/1
  q_d/1 -> MATLAB Function2/1(q)

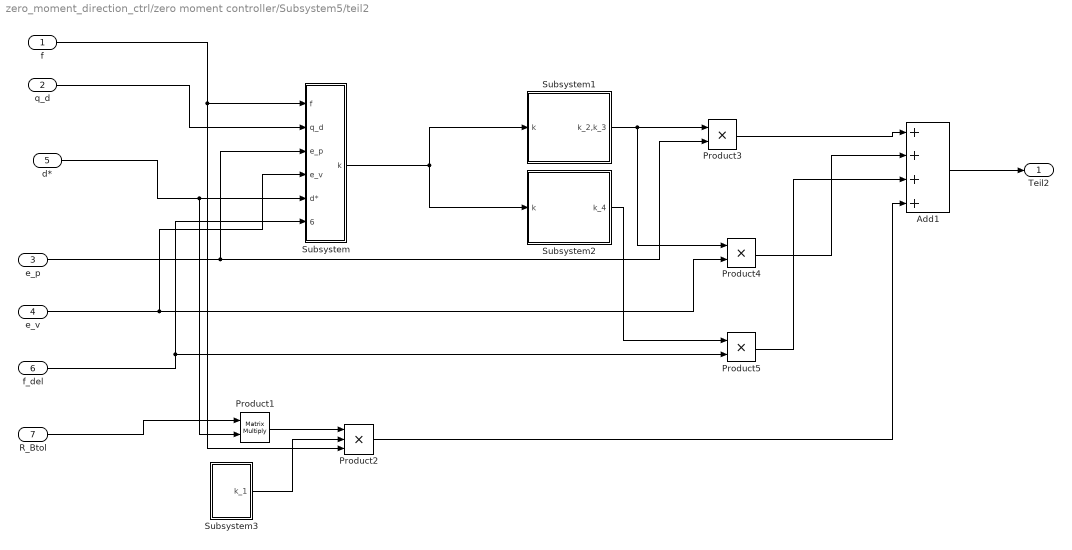
== system zero_moment_direction_ctrl/zero moment controller/Subsystem5/teil2 ==
  f : Inport
  q_d : Inport  Port=2
  e_p : Inport  Port=3
  e_v : Inport  Port=4
  d* : Inport  Port=5
  f_del : Inport  Port=6
  R_Btol : Inport  Port=7
  Add1 : Sum  Inputs=++++
  Product1 : Product  Multiplication=Matrix(*)
  Product2 : Product  Inputs=3
  Product3 : Product
  Product4 : Product
  Product5 : Product
  Subsystem : Subsystem
  Subsystem1 : Subsystem
  Subsystem2 : Subsystem
  Subsystem3 : Subsystem
  Teil2 : Outport
  wires:
  f/1 -> Product2/3, Subsystem/1(f)
  q_d/1 -> Subsystem/2(q_d)
  e_p/1 -> Product3/2, Subsystem/3(e_p)
  e_v/1 -> Product4/2, Subsystem/4(e_v)
  d*/1 -> Product1/2, Subsystem/5(d*)
  f_del/1 -> Product5/2, Subsystem/6(f_del)
  Subsystem/1(k) -> Subsystem1/1(k), Subsystem2/1(k)
  R_Btol/1 -> Product1/1
  Product1/1 -> Product2/1
  Subsystem3/1(k_1) -> Product2/2
  Subsystem1/1(k_2,k_3) -> Product4/1, Product3/1
  Product3/1 -> Add1/1
  Subsystem2/1(k_4) -> Product5/1
  Product4/1 -> Add1/2
  Product5/1 -> Add1/3
  Product2/1 -> Add1/4
  Add1/1 -> Teil2/1

== system zero_moment_direction_ctrl/zero moment controller/generate b2 and F2k/compute true Coupling Matrices ==
  Constant : Constant  Value=alpha_0
  Constant2 : Constant  Value=beta_0
  Constant3 : Constant  Value=k_0
  Constant4 : Constant  Value=L_0
  Constant5 : Constant  Value=b_0
  MATLAB Function5 : MATLAB Function  TreatAsAtomicUnit=on
  MATLAB Function6 : MATLAB Function  TreatAsAtomicUnit=on
  To Workspace : ToWorkspace  VariableName=yout  SampleTime=-1
      settings: Save2DSignal=2-D array (concatenate along first dimension)
  To Workspace1 : ToWorkspace  VariableName=yout1  SampleTime=-1
      settings: Save2DSignal=2-D array (concatenate along first dimension)
  F : Outport
  H : Outport  Port=2
  wires:
  MATLAB Function5/6(e_r6) -> MATLAB Function6/6(e_r6)
  Constant4/1 -> MATLAB Function6/9(L)
  MATLAB Function5/2(e_r2) -> MATLAB Function6/2(e_r2)
  MATLAB Function5/3(e_r3) -> MATLAB Function6/3(e_r3)
  MATLAB Function5/4(e_r4) -> MATLAB Function6/4(e_r4)
  MATLAB Function5/1(e_r1) -> MATLAB Function6/1(e_r1)
  MATLAB Function5/5(e_r5) -> MATLAB Function6/5(e_r5)
  Constant3/1 -> MATLAB Function6/8(k)
  Constant2/1 -> MATLAB Function5/2(beta)
  Constant/1 -> MATLAB Function5/1(alpha)
  Constant5/1 -> MATLAB Function6/7(b)
  MATLAB Function6/2(H) -> To Workspace/1, H/1
  MATLAB Function6/1(F) -> To Workspace1/1, F/1

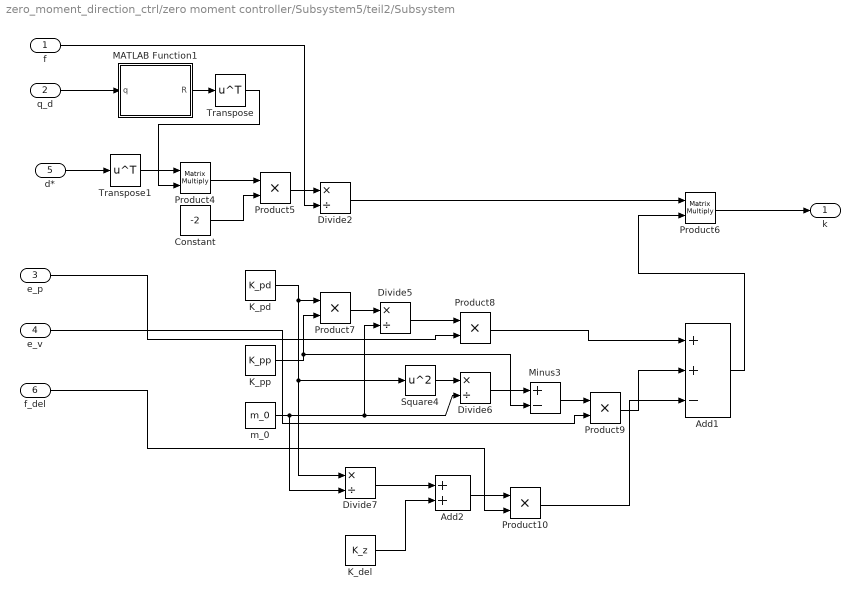
== system zero_moment_direction_ctrl/zero moment controller/Subsystem5/teil2/Subsystem ==
  f : Inport
  q_d : Inport  Port=2
  e_p : Inport  Port=3
  e_v : Inport  Port=4
  d* : Inport  Port=5
  f_del : Inport  Port=6
  Add1 : Sum  Inputs=++-
  Add2 : Sum
  Constant : Constant  Value=-2
  Divide{2,5..7} (4 alike) : Product  Inputs=*/
  K_del : Constant  Value=K_z
  K_pd : Constant  Value=K_pd
  K_pp : Constant  Value=K_pp
  MATLAB Function1 : MATLAB Function  TreatAsAtomicUnit=on
  Minus3 : Sum  Inputs=+-
  Product{5,7..10} (5 alike) : Product
  Product4 : Product  Multiplication=Matrix(*)
  Product6 : Product  Multiplication=Matrix(*)
  Square4 : Math  Operator=square  SaturateOnIntegerOverflow=on
  Transpose : Math  Operator=transpose  SaturateOnIntegerOverflow=on
  Transpose1 : Math  Operator=transpose  SaturateOnIntegerOverflow=on
  m_0 : Constant  Value=m_0
  k : Outport
  wires:
  K_pd/1 -> Divide7/1, Square4/1, Product7/1
  Divide2/1 -> Product6/1
  q_d/1 -> MATLAB Function1/1(q)
  Divide6/1 -> Minus3/1
  f/1 -> Divide2/2
  Transpose/1 -> Product4/2
  Transpose1/1 -> Product4/1
  K_pp/1 -> Product7/2, Minus3/2
  m_0/1 -> Divide7/2, Divide6/2, Divide5/2
  Constant/1 -> Product5/2
  Minus3/1 -> Product9/1
  Divide7/1 -> Add2/1
  K_del/1 -> Add2/2
  Square4/1 -> Divide6/1
  Add1/1 -> Product6/2
  Add2/1 -> Product10/1
  Product4/1 -> Product5/1
  Product5/1 -> Divide2/1
  Product7/1 -> Divide5/1
  Product6/1 -> k/1
  e_v/1 -> Product9/2
  f_del/1 -> Product10/2
  Product10/1 -> Add1/3
  Divide5/1 -> Product8/1
  Product8/1 -> Add1/1
  e_p/1 -> Product8/2
  d*/1 -> Transpose1/1
  Product9/1 -> Add1/2
  MATLAB Function1/1(R) -> Transpose/1

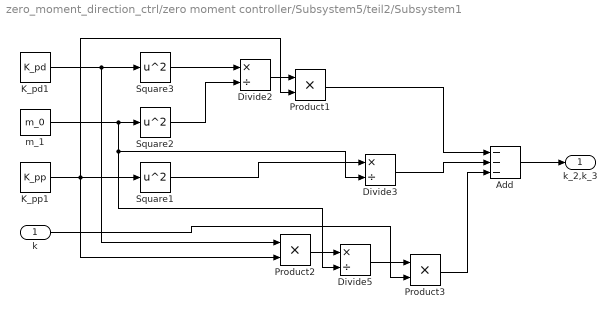
== system zero_moment_direction_ctrl/zero moment controller/Subsystem5/teil2/Subsystem1 ==
  k : Inport
  Add : Sum  Inputs=---
  Divide2 : Product  Inputs=*/
  Divide3 : Product  Inputs=*/
  Divide5 : Product  Inputs=*/
  K_pd1 : Constant  Value=K_pd
  K_pp1 : Constant  Value=K_pp
  Product1 : Product
  Product2 : Product
  Product3 : Product
  Square1 : Math  Operator=square  SaturateOnIntegerOverflow=on
  Square2 : Math  Operator=square  SaturateOnIntegerOverflow=on
  Square3 : Math  Operator=square  SaturateOnIntegerOverflow=on
  m_1 : Constant  Value=m_0
  k_2,k_3 : Outport
  wires:
  Square3/1 -> Divide2/1
  K_pp1/1 -> Product1/2, Product2/2, Square1/1
  m_1/1 -> Divide5/2, Divide3/2, Square2/1
  Square2/1 -> Divide2/2
  K_pd1/1 -> Product2/1, Square3/1
  Divide2/1 -> Product1/1
  Square1/1 -> Divide3/1
  Product2/1 -> Divide5/1
  Divide5/1 -> Product3/1
  k/1 -> Product3/2
  Product1/1 -> Add/1
  Divide3/1 -> Add/2
  Product3/1 -> Add/3
  Add/1 -> k_2,k_3/1

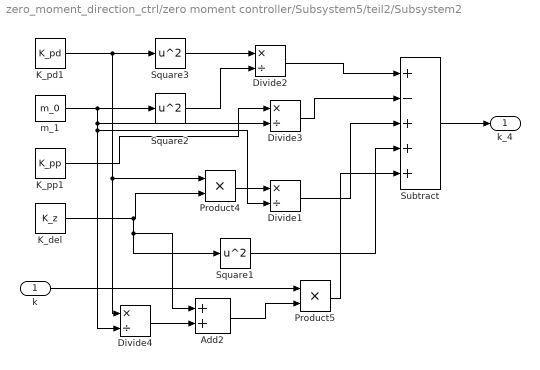
== system zero_moment_direction_ctrl/zero moment controller/Subsystem5/teil2/Subsystem2 ==
  k : Inport
  Add2 : Sum
  Divide{1..4} (4 alike) : Product  Inputs=*/
  K_del : Constant  Value=K_z
  K_pd1 : Constant  Value=K_pd
  K_pp1 : Constant  Value=K_pp
  Product4 : Product
  Product5 : Product
  Square1 : Math  Operator=square  SaturateOnIntegerOverflow=on
  Square2 : Math  Operator=square  SaturateOnIntegerOverflow=on
  Square3 : Math  Operator=square  SaturateOnIntegerOverflow=on
  Subtract : Sum  Inputs=+-+++
  m_1 : Constant  Value=m_0
  k_4 : Outport
  wires:
  Square3/1 -> Divide2/1
  K_pp1/1 -> Divide3/1
  m_1/1 -> Divide4/2, Divide1/2, Divide3/2, Square2/1
  Square2/1 -> Divide2/2
  K_pd1/1 -> Product4/1, Divide4/1, Square3/1
  Divide2/1 -> Subtract/1
  Divide3/1 -> Subtract/2
  K_del/1 -> Add2/1, Square1/1, Product4/2
  Product4/1 -> Divide1/1
  Divide1/1 -> Subtract/3
  Square1/1 -> Subtract/4
  k/1 -> Product5/1
  Divide4/1 -> Add2/2
  Add2/1 -> Product5/2
  Product5/1 -> Subtract/5
  Subtract/1 -> k_4/1

== system zero_moment_direction_ctrl/zero moment controller/Subsystem5/teil2/Subsystem3 ==
  Divide2 : Product  Inputs=*/
  Divide3 : Product  Inputs=*/
  K_pd1 : Constant  Value=K_pd
  K_pp1 : Constant  Value=K_pp
  Minus2 : Sum  Inputs=+-
  Square2 : Math  Operator=square  SaturateOnIntegerOverflow=on
  Square3 : Math  Operator=square  SaturateOnIntegerOverflow=on
  m_1 : Constant  Value=m_0
  k_1 : Outport
  wires:
  Square3/1 -> Divide2/1
  K_pp1/1 -> Divide3/1
  m_1/1 -> Divide3/2, Square2/1
  Square2/1 -> Divide2/2
  Minus2/1 -> k_1/1
  Divide2/1 -> Minus2/1
  K_pd1/1 -> Square3/1
  Divide3/1 -> Minus2/2

== matlab function zero_moment_direction_ctrl/zero moment controller/Subsystem5/MATLAB Function ==
  data: q input; R output
function R= quat2Dcm(q)
q1=q(1);
q2=q(2);
q3=q(3);
q4=q(4);
skew_w=[0 -q3 q2;
        q3 0 -q1
       -q2 q1 0];
R=eye(3)+2*q4*skew_w +2*(skew_w*skew_w);

== matlab function zero_moment_direction_ctrl/zero moment controller/Subsystem3/MATLAB Function16 ==
  data: omega input; w_x output
function w_x = omegaSkew3D(omega)

w_x = [0 -omega(3) omega(2);
        omega(3) 0 -omega(1);
        -omega(2) omega(1) 0];

== matlab function zero_moment_direction_ctrl/MATLAB Function4 ==
  data: R input; eul output
function eul = DCM2Euler(R)

%Roll
phi = atan2d(R(3,2),R(3,3));

%Pitch
psi = atan2d(-R(3,1),sqrt(R(1,1)^2 + R(2,1)^2));

%Yaw
gamma = atan2d(R(2,1),R(1,1));

eul=[phi;psi;gamma];

== matlab function zero_moment_direction_ctrl/compute true Coupling Matrices/MATLAB Function5 ==
  data: e_r1 output; e_r2 output; e_r3 output; e_r4 output; e_r5 output; e_r6 output; alpha input; beta input
function [e_r1, e_r2, e_r3, e_r4, e_r5, e_r6] = computeThrustDirections(alpha, beta)

e_r = zeros(3,6);
for it = 1:6
    alpha_i = alpha(it);
    beta_i = beta(it);
    gamma_i = (it-1)*pi/3 - pi/6;
    ca = cos(alpha_i);
    sa = sin(alpha_i);
    cb = cos(beta_i);
    sb = sin(beta_i);
    cy = cos(gamma_i);
    sy = sin(gamma_i);
    
    e_r(:,it) = [ca*sb*cy + sa*sy;
                ca*sb*sy - sa*cy;
                ca*cb];
            
end

e_r1 = e_r(:,1);
e_r2 = e_r(:,2);
e_r3 = e_r(:,3);
e_r4 = e_r(:,4);
e_r5 = e_r(:,5);
e_r6 = e_r(:,6);

== matlab function zero_moment_direction_ctrl/compute true Coupling Matrices/MATLAB Function6 ==
  data: F output; e_r1 input; e_r2 input; e_r3 input; e_r4 input; e_r5 input; e_r6 input; b input; k input; L input; H output
function [F,H]= computeCouplingMatrix(e_r1, e_r2, e_r3, e_r4, e_r5, e_r6, b, k, L)
% u = w^2

F = zeros(3,6);
H = zeros(3,6);

e_r = [e_r1 e_r2 e_r3 e_r4 e_r5 e_r6];

for it = 1:6
    gamma_i = (it-1)*pi/3 - pi/6;
   
    % thrust direction
    e_ri = e_r(:,it);
    
    % rotor position vector
    r_Ti =  L * [cos(gamma_i);
            sin(gamma_i);
            0];
        
    % Thrust force
    F(:,it) = k*e_ri;   
    
    % thrust and drag moment
    H(:,it) = k * cross(r_Ti, e_ri) + b * (-1)^(it-1) * e_ri;
    

    
end

== matlab function zero_moment_direction_ctrl/DC Motor Dynamics /MATLAB Function2 ==
  data: u input; y output
function y = fcn(u)

y = sqrt(abs(u))*sign(u);

== matlab function zero_moment_direction_ctrl/Motion Equations, quaternion/rotational Motion/MATLAB Function15 ==
  data: I input; I_inv output
function I_inv = inverse(I)

I_inv = inv(I);

== matlab function zero_moment_direction_ctrl/Motion Equations, quaternion/MATLAB Function ==
  data: q input; R output
function R= quat2Dcm(q)
q1=q(1);
q2=q(2);
q3=q(3);
q4=q(4);
skew_w=[0 -q3 q2;
        q3 0 -q1
       -q2 q1 0];
R=eye(3)+2*q4*skew_w +2*(skew_w*skew_w);

== matlab function zero_moment_direction_ctrl/zero moment controller/Subsystem4/MATLAB Function ==
  data: p input; y output; q input
function y = QuatCrossProduct(p, q)
p1=p(1);
p2=p(2);
p3=p(3);
p4=p(4);
q1=q(1);
q2=q(2);
q3=q(3);
q4=q(4);
M_p=[p4 -p3 p2 p1;
     p3 p4 -p1 p2;
     -p2 p1 p4 p3;
     -p1 -p2 -p3 p4];
y=M_p*q;

== matlab function zero_moment_direction_ctrl/zero moment controller/generate b2 and F2k/MATLAB Function ==
  data: F input; b2 output; H input; d input
function b2 = compute_b2 (F, H, d )
%  generate by by F, H, d*.
%  d*=F1*b2 
%  0=F2*b2
b2=[F; H]\[d; 0; 0; 0];

== matlab function zero_moment_direction_ctrl/zero moment controller/generate b2 and F2k/MATLAB Function3 ==
  data: d input; dnorm output
function dnorm = fcn(d)

dnorm=sqrt(d(1)^2+d(2)^2+d(3)^2);

== matlab function zero_moment_direction_ctrl/zero moment controller/MATLAB Function3 ==
  data: d input; dnorm output
function dnorm = fcn(d)

dnorm=sqrt(d(1)^2+d(2)^2+d(3)^2);

== matlab function zero_moment_direction_ctrl/zero moment controller/Subsystem5/teil1/MATLAB Function1 ==
  data: omega input; w_x output
function w_x = omegaSkew3D(omega)

w_x = [0 -omega(3) omega(2);
        omega(3) 0 -omega(1);
        -omega(2) omega(1) 0];

== matlab function zero_moment_direction_ctrl/zero moment controller/generate b2 and F2k/MATLAB Function1 ==
  data: V input; M_k output; M input
function M_k = compute_Mk(V, M)
%F2k:right pseudo-inverse of F2.
%F1*F2k=0
%F2*F2k=I
K=V;
M_k= K*M'/(M*K*M')  ;

== matlab function zero_moment_direction_ctrl/zero moment controller/generate b2 and F2k/MATLAB Function2 ==
  data: F input; V output; Vup input
function V = generateNullSpace_F1(F, Vup)
V=zeros(6,6);
for it=1:6
Vup_i=Vup(:, it);
Vdown_i =(F(: , 4:6 ))\(-F( : ,1:3)*Vup_i);
V_i=[Vup_i;Vdown_i];


V(:,it)=V_i;
end

== matlab function zero_moment_direction_ctrl/zero moment controller/generate b2 and F2k/compute true Coupling Matrices/MATLAB Function5 ==
  data: e_r1 output; e_r2 output; e_r3 output; e_r4 output; e_r5 output; e_r6 output; alpha input; beta input
function [e_r1, e_r2, e_r3, e_r4, e_r5, e_r6] = computeThrustDirections(alpha, beta)

e_r = zeros(3,6);
for it = 1:6
    alpha_i = alpha(it);
    beta_i = beta(it);
    gamma_i = (it-1)*pi/3 - pi/6;
    ca = cos(alpha_i);
    sa = sin(alpha_i);
    cb = cos(beta_i);
    sb = sin(beta_i);
    cy = cos(gamma_i);
    sy = sin(gamma_i);
    
    e_r(:,it) = [ca*sb*cy + sa*sy;
                ca*sb*sy - sa*cy;
                ca*cb];
            
end

e_r1 = e_r(:,1);
e_r2 = e_r(:,2);
e_r3 = e_r(:,3);
e_r4 = e_r(:,4);
e_r5 = e_r(:,5);
e_r6 = e_r(:,6);

== matlab function zero_moment_direction_ctrl/zero moment controller/Subsystem1/MATLAB Function1 ==
  data: q input; R output
function R= quat2Dcm(q)
q1=q(1);
q2=q(2);
q3=q(3);
q4=q(4);
skew_w=[0 -q3 q2;
        q3 0 -q1
       -q2 q1 0];
R=eye(3)+2*q4*skew_w +2*(skew_w*skew_w);

== matlab function zero_moment_direction_ctrl/DC Motor Dynamics /MATLAB Function3 ==
  data: u input; y output
function y = fcn(u)

y = u^2*sign(u);

== matlab function zero_moment_direction_ctrl/zero moment controller/generate b2 and F2k/compute true Coupling Matrices/MATLAB Function6 ==
  data: F output; e_r1 input; e_r2 input; e_r3 input; e_r4 input; e_r5 input; e_r6 input; b input; k input; L input; H output
function [F,H]= computeCouplingMatrix(e_r1, e_r2, e_r3, e_r4, e_r5, e_r6, b, k, L)
% u = w^2

F = zeros(3,6);
H = zeros(3,6);

e_r = [e_r1 e_r2 e_r3 e_r4 e_r5 e_r6];

for it = 1:6
    gamma_i = (it-1)*pi/3 - pi/6;
   
    % thrust direction
    e_ri = e_r(:,it);
    
    % rotor position vector
    r_Ti =  L * [cos(gamma_i);
            sin(gamma_i);
            0];
        
    % Thrust force
    F(:,it) = k*e_ri;   
    
    % thrust and drag moment
    H(:,it) = k * cross(r_Ti, e_ri) + b * (-1)^(it-1) * e_ri;
    

    
end

== matlab function zero_moment_direction_ctrl/zero moment controller/Subsystem4/MATLAB Function1 ==
  data: w input; y output
function y = omega2quat(w)
y=[w;0];

== matlab function zero_moment_direction_ctrl/zero moment controller/Subsystem6/MATLAB Function ==
  data: q input; y output
function y = quatInverse(q)
q1=q(1);
q2=q(2);
q3=q(3);
q4=q(4);
y = [-q1 -q2 -q3 q4]';

== matlab function zero_moment_direction_ctrl/zero moment controller/Subsystem5/teil2/Subsystem/MATLAB Function1 ==
  data: q input; R output
function R= quat2Dcm(q)
q1=q(1);
q2=q(2);
q3=q(3);
q4=q(4);
skew_w=[0 -q3 q2;
        q3 0 -q1
       -q2 q1 0];
R=eye(3)+2*q4*skew_w +2*(skew_w*skew_w);

== matlab function zero_moment_direction_ctrl/zero moment controller/Subsystem3/MATLAB Function1 ==
  data: q input; R output
function R= quat2Dcm(q)
q1=q(1);
q2=q(2);
q3=q(3);
q4=q(4);
skew_w=[0 -q3 q2;
        q3 0 -q1
       -q2 q1 0];
R=eye(3)+2*q4*skew_w +2*(skew_w*skew_w);

== matlab function zero_moment_direction_ctrl/zero moment controller/MATLAB Function1 ==
  data: R input; q output
function q   = DCM2Quat(R)

%%%%%%%%%%%%%%%%%%%%%%%%%%%%%%%%%%%%%%%%%%%%%%%%%%%%%%%%%%%%%%%%%%%%%%%%%%%
%
% M-file: Tool_DCM2Quat
%         -> impelmeted as M-Function
% Author: Marcel Tkocz
% Version: 27.01.2008
%
% Description:
%   This Function converts roll-pitch-yaw angels into their quaternion
%   equivalents.
%
% Inputs:
%   Orientation ... orientation in roll-pitch-yaw angels
%
% Outputs:
%   q           ... orientation in quaternions
%   
%%%%%%%%%%%%%%%%%%%%%%%%%%%%%%%%%%%%%%%%%%%%%%%%%%%%%%%%%%%%%%%%%%%%%%%%%%%

%--------------------------------------------------------------------------
% Calculation of Quaternions based on q1
%--------------------------------------------------------------------------
q = [0 0 0 1]';

if (1 + R(1,1) - R(2,2) - R(3,3)) > 0 
    q1 = 1/2*sqrt(1 + R(1,1) - R(2,2) - R(3,3));
    q2 = 1/(4*q1)*( R(1,2) + R(2,1));
    q3 = 1/(4*q1)*( R(1,3) + R(3,1));
    q4 = 1/(4*q1)*(-R(2,3) + R(3,2));

    if round(q1) ~= 0
        q = [q1; q2; q3; q4];
    end
end

%--------------------------------------------------------------------------
% Calculation of Quaternions based on q2
%--------------------------------------------------------------------------

if (1 - R(1,1) + R(2,2) - R(3,3)) > 0
    q2 = 1/2*sqrt(1 - R(1,1) + R(2,2) - R(3,3));
    q1 = 1/(4*q2)*( R(1,2) + R(2,1));
    q3 = 1/(4*q2)*( R(2,3) + R(3,2));
    q4 = 1/(4*q2)*( R(1,3) - R(3,1));

    if round(q2) ~= 0
        q = [q1; q2; q3; q4];
    end
end

%--------------------------------------------------------------------------
% Calculation of Quaternions based on q3
%--------------------------------------------------------------------------

if (1 - R(1,1) - R(2,2) + R(3,3)) > 0
    q3 = 1/2*sqrt(1 - R(1,1) - R(2,2) + R(3,3));
    q1 = 1/(4*q3)*( R(1,3) + R(3,1));
    q2 = 1/(4*q3)*( R(2,3) + R(3,2));
    q4 = 1/(4*q3)*(-R(1,2) + R(2,1));

    if round(q3) ~= 0
        q = [q1; q2; q3; q4];
    end
end

%--------------------------------------------------------------------------
% Calculation of Quaternions based on q4
%--------------------------------------------------------------------------

if (1 + R(1,1) + R(2,2) + R(3,3)) > 0
    q4 = 1/2*sqrt(1 + R(1,1) + R(2,2) + R(3,3));
    q1 = 1/(4*q4)*(-R(2,3) + R(3,2));
    q2 = 1/(4*q4)*(-R(3,1) + R(1,3));
    q3 = 1/(4*q4)*(-R(1,2) + R(2,1));

    if round(q4) ~= 0
        q = [q1; q2; q3; q4];
    end
end


end

== matlab function zero_moment_direction_ctrl/zero moment controller/Subsystem6/MATLAB Function1 ==
  data: p input; y output; q input
function y = QuatCrossProduct(p, q)
p1=p(1);
p2=p(2);
p3=p(3);
p4=p(4);
q1=q(1);
q2=q(2);
q3=q(3);
q4=q(4);
M_p=[p4 -p3 p2 p1;
    p3 p4 -p1 p2;
    -p2 p1 p4 p3;
    -p1 -p2 -p3 p4];
y=M_p*[q1 q2 q3 q4]';

== matlab function zero_moment_direction_ctrl/zero moment controller/Subsystem5/teil1/MATLAB Function ==
  data: q input; R output
function R = Quat2Dcm(q)
q1=q(1) ;
q2=q(2) ;
q3=q(3) ;
q4=q(4) ;

R = [q1^2-q2^2-q3^2+q4^2, 2*(q1*q2-q3*q4), 2*(q1*q3+q2*q4);
    2*(q1*q2+q3*q4), -q1^2+q2^2-q3^2+q4^2 2*(q2*q3-q1*q4);
    2*(q1*q3-q2*q4), 2*(q2*q3+q1*q4), -q1^2-q2^2+q3^2+q4^2];

== matlab function zero_moment_direction_ctrl/zero moment controller/Subsystem5/teil1/MATLAB Function2 ==
  data: q input; R output
function R= quat2Dcm(q)
q1=q(1);
q2=q(2);
q3=q(3);
q4=q(4);
skew_w=[0 -q3 q2;
        q3 0 -q1
       -q2 q1 0];
R=eye(3)+2*q4*skew_w +2*(skew_w*skew_w);

== matlab function zero_moment_direction_ctrl/create Force1 ==
  data: t input; tau_ext output
function tau_ext = createmoment(t)

if (0<t)&&(t<10)
    tau_ext=[1;1;1];

    else
        tau_ext=[0;0;0];
end
end

== matlab function zero_moment_direction_ctrl/zero moment controller/Subsystem6/MATLAB Function2 ==
  data: q input; epsilon output; eta output
function [epsilon, eta] = quatSeperate(q)
eta=q(4);
epsilon=[q(1) q(2) q(3)]';

== matlab function zero_moment_direction_ctrl/Motion Equations, quaternion/rotational Motion/MATLAB Function3 ==
  data: p input; y output; q input
function y = QuatCrossProduct(p, q)
p1=p(1);
p2=p(2);
p3=p(3);
p4=p(4);
q1=q(1);
q2=q(2);
q3=q(3);
q4=q(4);
M_p=[p4 -p3 p2 p1;
    p3 p4 -p1 p2;
    -p2 p1 p4 p3;
    -p1 -p2 -p3 p4];
y=M_p*[q1 q2 q3 q4]';

== matlab function zero_moment_direction_ctrl/Motion Equations, quaternion/rotational Motion/MATLAB Function6 ==
  data: w input; y output
function y = omega2quat(w)
y=[w;0];

== matlab function zero_moment_direction_ctrl/create Force ==
  data: t input; f_ext output
function f_ext  = createforce(t)

if (0<t)&&(t<10)
    f_ext=[1;1;1];
%else if (10<t)&&(t<20)
%   f_ext=[5;5;5];
    else
        f_ext=[0;0;0];
    end
end

== matlab function zero_moment_direction_ctrl/state estimation/MATLAB Function1 ==
  data: R input; eul output
function eul = DCM2Euler(R)

%Roll
phi = atan2d(R(3,2),R(3,3));

%Pitch
psi = atan2d(-R(3,1),sqrt(R(1,1)^2 + R(2,1)^2));

%Yaw
gamma = atan2d(R(2,1),R(1,1));

eul=[phi;psi;gamma];

== matlab function zero_moment_direction_ctrl/state estimation/MATLAB Function ==
  data: rpy input; R output
function R = Euler2DCM(rpy)
alpha = rpy(1);
beta = rpy(2);
gamma = rpy(3);

cg = cosd(gamma);
cb = cosd(beta);
sg = sind(gamma);
sb = sind(beta);
sa = sind(alpha);
ca = cosd(alpha);

R = [cg*cb, cg*sb*sa-sg*ca, cg*sb*ca+sg*sa;
    sg*cb, sg*sb*sa+cg*ca, sg*sb*ca-cg*sa;
    -sb, cb*sa, cb*ca];

== matlab function zero_moment_direction_ctrl/DC Motor Dynamics /MATLAB Function4 ==
  data: u input; y output
function y = fcn(u)

y = sqrt(abs(u))*sign(u);

== matlab function zero_moment_direction_ctrl/DC Motor Dynamics /MATLAB Function5 ==
  data: u input; y output
function y = fcn(u)

y = sqrt(abs(u))*sign(u);

== matlab function zero_moment_direction_ctrl/DC Motor Dynamics /MATLAB Function6 ==
  data: u input; y output; upper_limit input; lower_limit input
function y = fcn(u, upper_limit, lower_limit)

y = u^2*sign(u);

% set rotor velocities to limits in case of exceed
y(y>upper_limit) = upper_limit;
y(y<lower_limit) = lower_limit;
